simulink model "Resetmdl"  (R2013a)
settings: Solver=ode1  StartTime=0.0  StopTime=1  RelTol=1e-3
settings Model: SimulationMode=external  Creator=uqmech  LastModifiedBy=s4357594
settings DataIOCC: SignalLoggingSaveFormat=ModelDataLogs  SignalLoggingName=sigsOut
settings OptimizationCC: InitFltsAndDblsToZero=on
settings DebuggingCC: SaveWithParameterizedLinksMsg=none  SignalResolutionControl=TryResolveAllWithWarning  SolverPrmCheckMsg=none  MultiTaskDSMMsg=warning  MultiTaskCondExecSysMsg=none  StrictBusMsg=None
settings RTWCC: SystemTargetFile=rtwin.tlc  TemplateMakefile=rtwin.tmf  Description=Real-Time Windows Target  ProcessScript=rtwin_make_rtw_hook  IncludeERTFirstTime=on
settings RTWinTargetCC: TargetFcnLib=ansi_tfl_tmw.mat  TargetLibSuffix=_rtwin.lib  TargetPreCompLibLocation=C:\Program Files\MATLAB\R2013a\toolbox\rtw\targets\rtwin\lib\win64  CodeReplacementLibrary=ANSI_C  ModelReferenceCompliant=off  CompOptLevelCompliant=off  RTWinDir=C:/PROGRA~1/MATLAB/R2013a/toolbox/rtw/targets/rtwin  TargetArch=win64

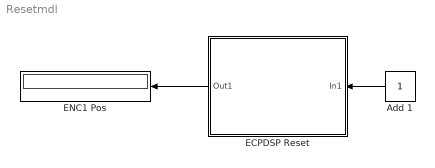
== system Resetmdl ==
  Add 1 : Constant
  ECPDSP Reset : Subsystem  mask{BaseAddr='0xC000', STime=0.001, TimeOutPer=500, HWAccess=on}
      mask prompts: BaseAddr "Base I/O Address"; STime "Sample Time (Sec)"; TimeOutPer "Timeout Period (500 ~ 2000)"; HWAccess "Hardware Access"
      mask Display: color('black');disp('ECPDSP Reset\n Will reset Dacs and Encs')
  ENC1 Pos : Display
  wires:
  Add 1/1 -> ECPDSP Reset/1(In1)
  ECPDSP Reset/1(Out1) -> ENC1 Pos/1

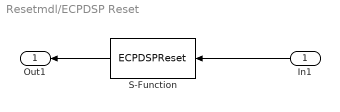
== system Resetmdl/ECPDSP Reset ==
  In1 : Inport
  S-Function : S-Function  FunctionName=ECPDSPReset  Parameters=BaseAddr,STime,TimeOutPer,HWAccess  EnableBusSupport=off
  Out1 : Outport
  wires:
  In1/1 -> S-Function/1
  S-Function/1 -> Out1/1
